simulink model "MOSSE_HDL_code_gen_final"  (Simulink 8.2)
settings: Solver=FixedStepDiscrete  SolverMode=SingleTasking  StartTime=0.0  StopTime=20*640*360  RelTol=1e-3
InitFcn:
  | %% DSPBuilder Start
  | alt_dspbuilder_update_model(bdroot)
  | %% DSPBuilder End
  | param
StopFcn:
  | % r = rcount.Data(:,:);
  | % w = wcount.Data(:,:);
  | % d = dout.Data(:,:);
  | % ir = read.Data(:,:);
  | % iw = write.Data(:,:);
  | % z = double([ir iw d r w]');
  | %logic_analyzer
values from neighbouring files (symbols this model uses):
  Gau = [4035 -3983 3832 -3589 3269 -2890 2472 -2039 1612 -1211 854 -553 ... (4096 elements, 1x4096)]    [Gauss_coeff.mat]    (also in param.m = reshape(conj(Gau'), 1, 4096))
undefined symbols (not defined in the file or in its folder): jet, psr, source_1, source_2, State_Machine, State_Transition_Table1, window_hann
libraries: allblocks_alteradspbuilder2 x182, hdldemolib x2, dspsigattribs x2, dspmtrx3 x2, visionsinks x1, visiontextngfix x1, dspvision x1
(part 3 of 3)

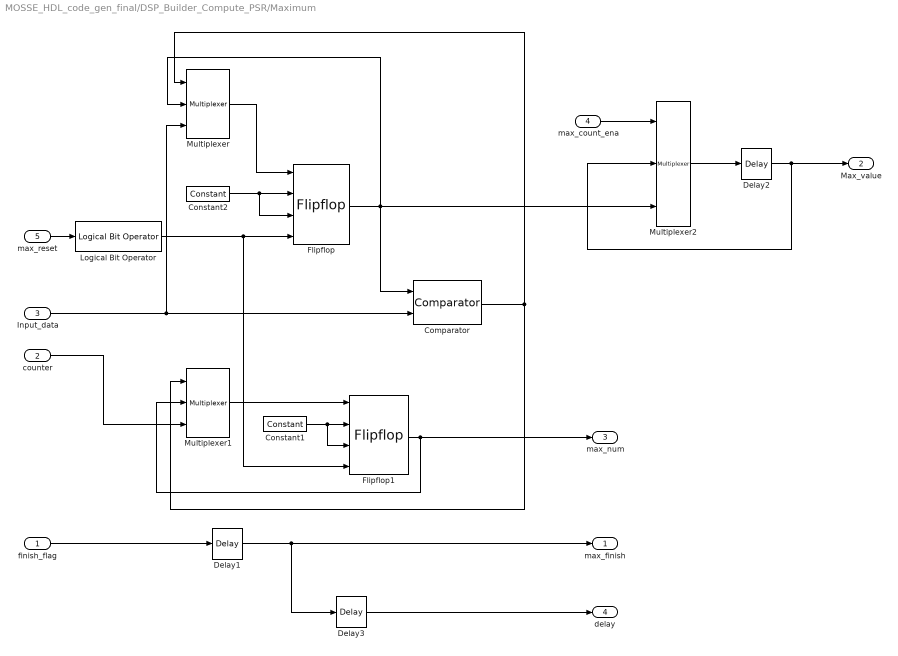
== system MOSSE_HDL_code_gen_final/DSP_Builder_Compute_PSR/Maximum ==
  finish_flag : Inport
  counter : Inport  Port=2
  Input_data : Inport  Port=3
  max_count_ena : Inport  Port=4
  max_reset : Inport  Port=5
  Comparator : allblocks_alteradspbuilder2/Comparator  direction=a < b  pipeline_display=0  allowFloatingPointOverride=on  logOutputs=off  logFile=d:\Project\AutoTracking\model\MOSSE_work\MOSSE_model\MOSSE_Final_models\tb_MOSSE_HDL_final\MOSSE%5FHDL%5Ffinal_DSP%5FBuilder%5FCompute%5FPSR_Maximum_Comparator.fixedpointlog
  Constant1 : allblocks_alteradspbuilder2/Constant  mask_cst=1  BusType=Single Bit  bwl=24  bwr=0  roundMode=Truncate  satMode=Wrap  SpecifyClock=off  allowFloatingPointOverride=on  logOutputs=off  logFile=d:\Project\AutoTracking\model\MOSSE_work\MOSSE_model\MOSSE_Final_models\tb_MOSSE_HDL_final\MOSSE%5FHDL%5Ffinal_DSP%5FBuilder%5FCompute%5FPSR_Maximum_Constant1.fixedpointlog
  Constant2 : allblocks_alteradspbuilder2/Constant  mask_cst=1  BusType=Single Bit  bwl=24  bwr=0  roundMode=Truncate  satMode=Wrap  SpecifyClock=off  allowFloatingPointOverride=on  logOutputs=off  logFile=d:\Project\AutoTracking\model\MOSSE_work\MOSSE_model\MOSSE_Final_models\tb_MOSSE_HDL_final\MOSSE%5FHDL%5Ffinal_DSP%5FBuilder%5FCompute%5FPSR_Maximum_Constant2.fixedpointlog
  Delay1 : allblocks_alteradspbuilder2/Delay  pipeline=2  pipeline_display=2  ClockPhase=1  use_ena=off  use_sclr=off  allowFloatingPointOverride=on  logOutputs=off  logFile=d:\Project\AutoTracking\model\MOSSE_work\MOSSE_model\MOSSE_Final_models\tb_MOSSE_HDL_final\MOSSE%5FHDL%5Ffinal_DSP%5FBuilder%5FCompute%5FPSR_Maximum_Delay1.fixedpointlog  use_init=off  reset_value=1
  Delay2 : allblocks_alteradspbuilder2/Delay  pipeline=1  pipeline_display=1  ClockPhase=1  use_ena=off  use_sclr=off  allowFloatingPointOverride=on  logOutputs=off  logFile=d:\Project\AutoTracking\model\MOSSE_work\MOSSE_model\MOSSE_Final_models\tb_MOSSE_HDL_final\MOSSE%5FHDL%5Ffinal_DSP%5FBuilder%5FCompute%5FPSR_Maximum_Delay2.fixedpointlog  use_init=off  reset_value=1
  Delay3 : allblocks_alteradspbuilder2/Delay  pipeline=1  pipeline_display=1  ClockPhase=1  use_ena=off  use_sclr=off  allowFloatingPointOverride=on  logOutputs=off  logFile=d:\Project\AutoTracking\model\MOSSE_work\MOSSE_model\MOSSE_Final_models\tb_MOSSE_HDL_final\MOSSE%5FHDL%5Ffinal_DSP%5FBuilder%5FCompute%5FPSR_Maximum_Delay3.fixedpointlog  use_init=off  reset_value=1
  Flipflop : allblocks_alteradspbuilder2/Flipflop  mode=DFFE  BusType=Signed Integer  bwl=16  bwr=2  pipeline_display=1
  Flipflop1 : allblocks_alteradspbuilder2/Flipflop  mode=DFFE  BusType=Signed Integer  bwl=16  bwr=2  pipeline_display=1
  Logical Bit Operator : allblocks_alteradspbuilder2/Logical Bit Operator  LogicalOperator=NOT  user_inputs=2  pipeline_display=0
  Multiplexer : allblocks_alteradspbuilder2/Multiplexer  numInputs=2  pipeline=0  oneHot=off  pipeline_display=0  use_ena=off  use_aclr=off  allowFloatingPointOverride=on  logOutputs=off  logFile=d:\Project\AutoTracking\model\MOSSE_work\MOSSE_model\MOSSE_Final_models\tb_MOSSE_HDL_final\MOSSE%5FHDL%5Ffinal_DSP%5FBuilder%5FCompute%5FPSR_Maximum_Multiplexer.fixedpointlog
  Multiplexer1 : allblocks_alteradspbuilder2/Multiplexer  numInputs=2  pipeline=0  oneHot=off  pipeline_display=0  use_ena=off  use_aclr=off  allowFloatingPointOverride=on  logOutputs=off  logFile=d:\Project\AutoTracking\model\MOSSE_work\MOSSE_model\MOSSE_Final_models\tb_MOSSE_HDL_final\MOSSE%5FHDL%5Ffinal_DSP%5FBuilder%5FCompute%5FPSR_Maximum_Multiplexer1.fixedpointlog
  Multiplexer2 : allblocks_alteradspbuilder2/Multiplexer  numInputs=2  pipeline=0  oneHot=off  pipeline_display=0  use_ena=off  use_aclr=off  allowFloatingPointOverride=on  logOutputs=off  logFile=d:\Project\AutoTracking\model\MOSSE_work\MOSSE_model\MOSSE_Final_models\tb_MOSSE_HDL_final\MOSSE%5FHDL%5Ffinal_DSP%5FBuilder%5FCompute%5FPSR_Maximum_Multiplexer2.fixedpointlog
  max_finish : Outport
  Max_value : Outport  Port=2
  max_num : Outport  Port=3
  delay : Outport  Port=4
  wires:
  Comparator/1 -> Multiplexer/1, Multiplexer1/1
  Flipflop/1 -> Comparator/1, Multiplexer2/3, Multiplexer/2
  Multiplexer/1 -> Flipflop/1
  Constant2/1 -> Flipflop/3, Flipflop/2
  Input_data/1 -> Multiplexer/3, Comparator/2
  Flipflop1/1 -> max_num/1, Multiplexer1/2
  Multiplexer1/1 -> Flipflop1/1
  Constant1/1 -> Flipflop1/3, Flipflop1/2
  counter/1 -> Multiplexer1/3
  Delay1/1 -> max_finish/1, Delay3/1
  max_count_ena/1 -> Multiplexer2/1
  Multiplexer2/1 -> Delay2/1
  Delay2/1 -> Multiplexer2/2, Max_value/1
  Delay3/1 -> delay/1
  finish_flag/1 -> Delay1/1
  Logical Bit Operator/1 -> Flipflop1/4, Flipflop/4
  max_reset/1 -> Logical Bit Operator/1

== system MOSSE_HDL_code_gen_final/DSP_Builder_Compute_PSR/Mean1 ==
  finish_flag : Inport
  Input_data : Inport  Port=2
  mean_count_ena : Inport  Port=3
  mean_reset : Inport  Port=4
  Barrel Shifter : allblocks_alteradspbuilder2/Barrel Shifter  BusType=Signed Integer  bwl=32  bwr=8  pipeline=off  infer_distance=off  distance_length=4  ShiftDirection=Shift right  use_ena=off  use_aclr=off  UseDedicatedCircuitry=off  pipeline_display=0  allowFloatingPointOverride=on  logOutputs=off  logFile=d:\Project\AutoTracking\model\MOSSE_work\MOSSE_model\MOSSE_Final_models\tb_MOSSE_HDL_final\MOSSE%5FHDL%5Ffinal_DSP%5FBuilder%5FCompute%5FPSR_Mean1_Barrel+Shifter.fixedpointlog
  Constant2 : allblocks_alteradspbuilder2/Constant  mask_cst=12  BusType=Unsigned Integer  bwl=4  bwr=0  roundMode=Truncate  satMode=Wrap  SpecifyClock=off  allowFloatingPointOverride=on  logOutputs=off  logFile=d:\Project\AutoTracking\model\MOSSE_work\MOSSE_model\MOSSE_Final_models\tb_MOSSE_HDL_final\MOSSE%5FHDL%5Ffinal_DSP%5FBuilder%5FCompute%5FPSR_Mean1_Constant2.fixedpointlog
  Delay1 : allblocks_alteradspbuilder2/Delay  pipeline=1  pipeline_display=1  ClockPhase=1  use_ena=off  use_sclr=off  allowFloatingPointOverride=on  logOutputs=off  logFile=d:\Project\AutoTracking\model\MOSSE_work\MOSSE_model\MOSSE_Final_models\tb_MOSSE_HDL_final\MOSSE%5FHDL%5Ffinal_DSP%5FBuilder%5FCompute%5FPSR_Mean1_Delay1.fixedpointlog  use_init=off  reset_value=1
  Delay2 : allblocks_alteradspbuilder2/Delay  pipeline=1  pipeline_display=1  ClockPhase=1  use_ena=off  use_sclr=off  allowFloatingPointOverride=on  logOutputs=off  logFile=d:\Project\AutoTracking\model\MOSSE_work\MOSSE_model\MOSSE_Final_models\tb_MOSSE_HDL_final\MOSSE%5FHDL%5Ffinal_DSP%5FBuilder%5FCompute%5FPSR_Mean1_Delay2.fixedpointlog  use_init=off  reset_value=1
  Multiplexer2 : allblocks_alteradspbuilder2/Multiplexer  numInputs=2  pipeline=0  oneHot=off  pipeline_display=0  use_ena=off  use_aclr=off  allowFloatingPointOverride=on  logOutputs=off  logFile=d:\Project\AutoTracking\model\MOSSE_work\MOSSE_model\MOSSE_Final_models\tb_MOSSE_HDL_final\MOSSE%5FHDL%5Ffinal_DSP%5FBuilder%5FCompute%5FPSR_Mean1_Multiplexer2.fixedpointlog
  Pipelined Adder : allblocks_alteradspbuilder2/Pipelined Adder  BusType=Signed Integer  bwl=32  bwr=0  pipeline=1  pipeline_display=1  AddSubDirection=ADD  use_cin=off  use_ovl=off  use_addsub=off  use_ena=off  use_aclr=on  or_aclr_inputs=off
  mean_finish : Outport
  mean_value : Outport  Port=2
  wires:
  Constant2/1 -> Barrel Shifter/2
  Pipelined Adder/1 -> Pipelined Adder/1, Barrel Shifter/1
  Input_data/1 -> Pipelined Adder/2
  Barrel Shifter/1 -> Multiplexer2/3
  mean_count_ena/1 -> Multiplexer2/1
  Multiplexer2/1 -> Delay2/1
  Delay2/1 -> mean_value/1, Multiplexer2/2
  finish_flag/1 -> Delay1/1
  Delay1/1 -> mean_finish/1
  mean_reset/1 -> Pipelined Adder/3

== system MOSSE_HDL_code_gen_final/DSP_Builder_Compute_PSR/Psr1 ==
  max : Inport
  mean : Inport  Port=2
  std : Inport  Port=3
  psr_count_ena : Inport  Port=4
  std_finish : Inport  Port=5
  Delay1 : allblocks_alteradspbuilder2/Delay  pipeline=1  pipeline_display=1  ClockPhase=1  use_ena=off  use_sclr=off  allowFloatingPointOverride=on  logOutputs=off  logFile=d:\Project\AutoTracking\model\MOSSE_work\MOSSE_model\MOSSE_Final_models\tb_MOSSE_HDL_final\MOSSE%5FHDL%5Ffinal_DSP%5FBuilder%5FCompute%5FPSR_Psr1_Delay1.fixedpointlog  use_init=off  reset_value=1
  Delay2 : allblocks_alteradspbuilder2/Delay  pipeline=1  pipeline_display=1  ClockPhase=1  use_ena=off  use_sclr=off  allowFloatingPointOverride=on  logOutputs=off  logFile=d:\Project\AutoTracking\model\MOSSE_work\MOSSE_model\MOSSE_Final_models\tb_MOSSE_HDL_final\MOSSE%5FHDL%5Ffinal_DSP%5FBuilder%5FCompute%5FPSR_Psr1_Delay2.fixedpointlog  use_init=off  reset_value=1
  Divider : allblocks_alteradspbuilder2/Divider  BusType=Signed Integer  bwl=32  bwr=0  pipeline=0  pipeline_display=0  use_ena=off  use_aclr=off
  Multiplexer3 : allblocks_alteradspbuilder2/Multiplexer  numInputs=2  pipeline=0  oneHot=off  pipeline_display=0  use_ena=off  use_aclr=off  allowFloatingPointOverride=on  logOutputs=off  logFile=d:\Project\AutoTracking\model\MOSSE_work\MOSSE_model\MOSSE_Final_models\tb_MOSSE_HDL_final\MOSSE%5FHDL%5Ffinal_DSP%5FBuilder%5FCompute%5FPSR_Psr1_Multiplexer3.fixedpointlog
  Pipelined Adder : allblocks_alteradspbuilder2/Pipelined Adder  BusType=Signed Integer  bwl=32  bwr=0  pipeline=0  pipeline_display=0  AddSubDirection=SUB  use_cin=off  use_ovl=off  use_addsub=off  use_ena=off  use_aclr=off  or_aclr_inputs=on
  Psr_finish : Outport
  psr : Outport  Port=2
  wires:
  Pipelined Adder/1 -> Divider/1
  Divider/1 -> Multiplexer3/3
  max/1 -> Pipelined Adder/1
  mean/1 -> Pipelined Adder/2
  std/1 -> Divider/2
  psr_count_ena/1 -> Multiplexer3/1
  Multiplexer3/1 -> Delay2/1
  Delay2/1 -> psr/1, Multiplexer3/2
  std_finish/1 -> Delay1/1
  Delay1/1 -> Psr_finish/1

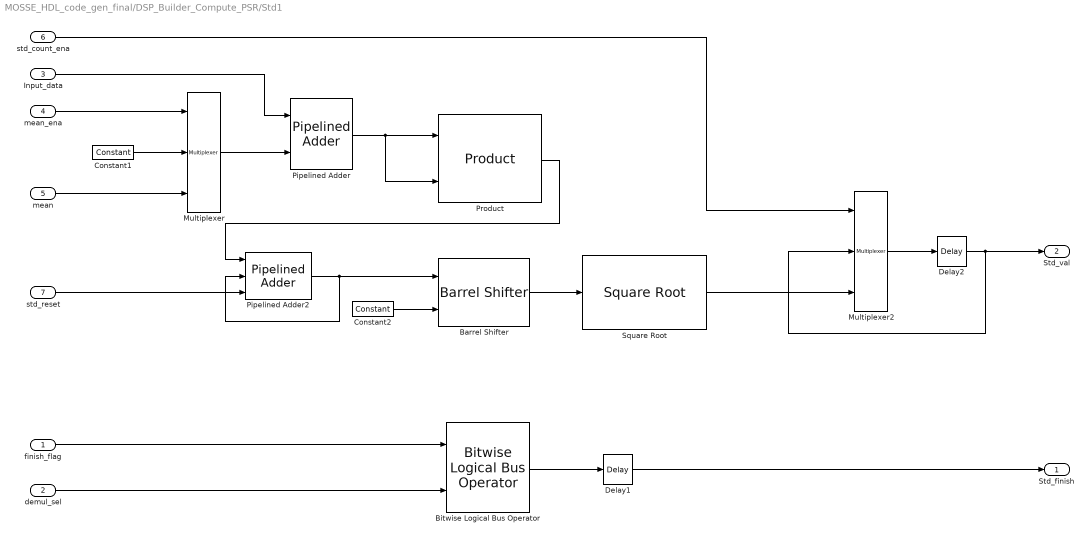
== system MOSSE_HDL_code_gen_final/DSP_Builder_Compute_PSR/Std1 ==
  finish_flag : Inport
  demul_sel : Inport  Port=2
  Input_data : Inport  Port=3
  mean_ena : Inport  Port=4
  mean : Inport  Port=5
  std_count_ena : Inport  Port=6
  std_reset : Inport  Port=7
  Barrel Shifter : allblocks_alteradspbuilder2/Barrel Shifter  BusType=Signed Integer  bwl=44  bwr=8  pipeline=off  infer_distance=off  distance_length=4  ShiftDirection=Shift right  use_ena=off  use_aclr=off  UseDedicatedCircuitry=off  pipeline_display=0  allowFloatingPointOverride=on  logOutputs=off  logFile=d:\Project\AutoTracking\model\MOSSE_work\MOSSE_model\MOSSE_Final_models\tb_MOSSE_HDL_final\MOSSE%5FHDL%5Ffinal_DSP%5FBuilder%5FCompute%5FPSR_Std1_Barrel+Shifter.fixedpointlog
  Bitwise Logical Bus Operator : allblocks_alteradspbuilder2/Bitwise Logical Bus Operator  BusType=Unsigned Integer  bwl=1  bwr=0  LogicalOperator=AND  pipeline_display=0
  Constant1 : allblocks_alteradspbuilder2/Constant  mask_cst=0  BusType=Signed Integer  bwl=32  bwr=0  roundMode=Truncate  satMode=Wrap  SpecifyClock=off  allowFloatingPointOverride=on  logOutputs=off  logFile=d:\Project\AutoTracking\model\MOSSE_work\MOSSE_model\MOSSE_Final_models\tb_MOSSE_HDL_final\MOSSE%5FHDL%5Ffinal_DSP%5FBuilder%5FCompute%5FPSR_Std1_Constant1.fixedpointlog
  Constant2 : allblocks_alteradspbuilder2/Constant  mask_cst=12  BusType=Unsigned Integer  bwl=4  bwr=0  roundMode=Truncate  satMode=Wrap  SpecifyClock=off  allowFloatingPointOverride=on  logOutputs=off  logFile=d:\Project\AutoTracking\model\MOSSE_work\MOSSE_model\MOSSE_Final_models\tb_MOSSE_HDL_final\MOSSE%5FHDL%5Ffinal_DSP%5FBuilder%5FCompute%5FPSR_Std1_Constant2.fixedpointlog
  Delay1 : allblocks_alteradspbuilder2/Delay  pipeline=1  pipeline_display=1  ClockPhase=1  use_ena=off  use_sclr=off  allowFloatingPointOverride=on  logOutputs=off  logFile=d:\Project\AutoTracking\model\MOSSE_work\MOSSE_model\MOSSE_Final_models\tb_MOSSE_HDL_final\MOSSE%5FHDL%5Ffinal_DSP%5FBuilder%5FCompute%5FPSR_Std1_Delay1.fixedpointlog  use_init=off  reset_value=1
  Delay2 : allblocks_alteradspbuilder2/Delay  pipeline=1  pipeline_display=1  ClockPhase=1  use_ena=off  use_sclr=off  allowFloatingPointOverride=on  logOutputs=off  logFile=d:\Project\AutoTracking\model\MOSSE_work\MOSSE_model\MOSSE_Final_models\tb_MOSSE_HDL_final\MOSSE%5FHDL%5Ffinal_DSP%5FBuilder%5FCompute%5FPSR_Std1_Delay2.fixedpointlog  use_init=off  reset_value=1
  Multiplexer : allblocks_alteradspbuilder2/Multiplexer  numInputs=2  pipeline=0  oneHot=off  pipeline_display=0  use_ena=off  use_aclr=off  allowFloatingPointOverride=on  logOutputs=off  logFile=d:\Project\AutoTracking\model\MOSSE_work\MOSSE_model\MOSSE_Final_models\tb_MOSSE_HDL_final\MOSSE%5FHDL%5Ffinal_DSP%5FBuilder%5FCompute%5FPSR_Std1_Multiplexer.fixedpointlog
  Multiplexer2 : allblocks_alteradspbuilder2/Multiplexer  numInputs=2  pipeline=0  oneHot=off  pipeline_display=0  use_ena=off  use_aclr=off  allowFloatingPointOverride=on  logOutputs=off  logFile=d:\Project\AutoTracking\model\MOSSE_work\MOSSE_model\MOSSE_Final_models\tb_MOSSE_HDL_final\MOSSE%5FHDL%5Ffinal_DSP%5FBuilder%5FCompute%5FPSR_Std1_Multiplexer2.fixedpointlog
  Pipelined Adder : allblocks_alteradspbuilder2/Pipelined Adder  BusType=Signed Integer  bwl=32  bwr=0  pipeline=0  pipeline_display=0  AddSubDirection=SUB  use_cin=off  use_ovl=off  use_addsub=off  use_ena=off  use_aclr=off  or_aclr_inputs=on
  Pipelined Adder2 : allblocks_alteradspbuilder2/Pipelined Adder  BusType=Signed Integer  bwl=44  bwr=0  pipeline=1  pipeline_display=1  AddSubDirection=ADD  use_cin=off  use_ovl=off  use_addsub=off  use_ena=off  use_aclr=on  or_aclr_inputs=off
  Product : allblocks_alteradspbuilder2/Product  BusType=Signed Integer  bwl=32  bwr=0  pipeline=0  pipeline_display=0  phase_selection=1  use_ena=off  use_aclr=off  UseLPM=off  UseDedicatedCircuitry=on  allowFloatingPointOverride=on  logOutputs=off  logFile=d:\Project\AutoTracking\model\MOSSE_work\MOSSE_model\MOSSE_Final_models\tb_MOSSE_HDL_final\MOSSE%5FHDL%5Ffinal_DSP%5FBuilder%5FCompute%5FPSR_Std1_Product.fixedpointlog
  Square Root : allblocks_alteradspbuilder2/Square Root  BusType=Unsigned Integer  bwl=44  bwr=0  pipeline=0  pipeline_display=0  use_remain=off  use_ena=off  use_aclr=off
  Std_finish : Outport
  Std_val : Outport  Port=2
  wires:
  Pipelined Adder/1 -> Product/2, Product/1
  Product/1 -> Pipelined Adder2/1
  Constant2/1 -> Barrel Shifter/2
  Pipelined Adder2/1 -> Pipelined Adder2/2, Barrel Shifter/1
  Barrel Shifter/1 -> Square Root/1
  Square Root/1 -> Multiplexer2/3
  Input_data/1 -> Pipelined Adder/1
  demul_sel/1 -> Bitwise Logical Bus Operator/2
  finish_flag/1 -> Bitwise Logical Bus Operator/1
  Delay1/1 -> Std_finish/1
  Constant1/1 -> Multiplexer/2
  mean_ena/1 -> Multiplexer/1
  mean/1 -> Multiplexer/3
  Multiplexer/1 -> Pipelined Adder/2
  std_count_ena/1 -> Multiplexer2/1
  Multiplexer2/1 -> Delay2/1
  Delay2/1 -> Std_val/1, Multiplexer2/2
  Bitwise Logical Bus Operator/1 -> Delay1/1
  std_reset/1 -> Pipelined Adder2/3

== system MOSSE_HDL_code_gen_final/DSP_Builder_Compute_PSR/Vals_gen ==
  count_ena : Inport
  counter : Inport  Port=2
  demul_sel : Inport  Port=3
  Constant2 : allblocks_alteradspbuilder2/Constant  mask_cst=0  BusType=Single Bit  bwl=16  bwr=0  roundMode=Truncate  satMode=Wrap  SpecifyClock=off  allowFloatingPointOverride=on  logOutputs=off  logFile=d:\Project\AutoTracking\model\MOSSE_work\MOSSE_model\MOSSE_Final_models\tb_MOSSE_HDL_final\MOSSE%5FHDL%5Ffinal_DSP%5FBuilder%5FCompute%5FPSR_Vals%5Fgen_Constant2.fixedpointlog
  Demultiplexer : allblocks_alteradspbuilder2/Demultiplexer  numOutputs=2  pipeline_display=1  use_ena=off  use_sclr=off  allowFloatingPointOverride=on  logOutputs=off  logFile=d:\Project\AutoTracking\model\MOSSE_work\MOSSE_model\MOSSE_Final_models\tb_MOSSE_HDL_final\MOSSE%5FHDL%5Ffinal_DSP%5FBuilder%5FCompute%5FPSR_Vals%5Fgen_Demultiplexer%3A%3Aq.fixedpointlog,d:\Project\AutoTracking\model\MOSSE_work\MOSSE_model\MOSSE_Final_models\tb_MOSSE_HDL_final\MOSSE%5FHDL%5Ffinal_DSP%5FBuilder%5FCompute%5FPSR_Vals%5Fgen_Demultiplexer%3A%3Aq.fixedpointlog,
  Multiplexer : allblocks_alteradspbuilder2/Multiplexer  numInputs=2  pipeline=0  oneHot=off  pipeline_display=0  use_ena=off  use_aclr=off  allowFloatingPointOverride=on  logOutputs=off  logFile=d:\Project\AutoTracking\model\MOSSE_work\MOSSE_model\MOSSE_Final_models\tb_MOSSE_HDL_final\MOSSE%5FHDL%5Ffinal_DSP%5FBuilder%5FCompute%5FPSR_Vals%5Fgen_Multiplexer.fixedpointlog
  1_channel : Outport
  2_channel : Outport  Port=2
  wires:
  Multiplexer/1 -> Demultiplexer/1
  Demultiplexer/1 -> 1_channel/1
  Demultiplexer/2 -> 2_channel/1
  demul_sel/1 -> Demultiplexer/2
  Constant2/1 -> Multiplexer/2
  counter/1 -> Multiplexer/3
  count_ena/1 -> Multiplexer/1

== system MOSSE_HDL_code_gen_final/DSP_Builder_Mult_complex/Gauss_table ==
  rst : Inport
  enb : Inport  Port=2
  Counter : allblocks_alteradspbuilder2/Counter  BusType=Unsigned Integer  bwl=12  bwr=0  use_modulo=off  modulo=255  SpecifyClock=off  direction=Increment  use_sload=off  use_sset=off  svalue=1  use_clk_ena=off  use_ena=on  use_sclr=on  pipeline_display=1
  ROM : allblocks_alteradspbuilder2/ROM  numwords=4096  BusType=Signed Integer  bwl=16  bwr=0  memory_type=AUTO  ram_type=ROM  initialization=From MATLAB array  init_file=input.hex  init_array=imag(Gau)  register_outputs=off  use_ena=off  ClockPhase=1  pipeline_display=1  allowFloatingPointOverride=on  logOutputs=off  logFile=E:\Project\AutoTracking\AutoTrack\Model\MOSSE_algorithm\MOSSE_simulink\tb_MOSSE_HDL_code_gen_final\MOSSE%5FHDL%5Fcode%5Fgen%5Ffinal_DSP%5FBuilder%5FMult%5Fcomplex_Gauss%5Ftable_ROM.fixedpointlog  enable_runtime_mod=off  instance_name=AAAA
  ROM1 : allblocks_alteradspbuilder2/ROM  numwords=4096  BusType=Signed Integer  bwl=16  bwr=0  memory_type=AUTO  ram_type=ROM  initialization=From MATLAB array  init_file=input.hex  init_array=real(Gau)  register_outputs=off  use_ena=off  ClockPhase=1  pipeline_display=1  allowFloatingPointOverride=on  logOutputs=off  logFile=E:\Project\AutoTracking\AutoTrack\Model\MOSSE_algorithm\MOSSE_simulink\tb_MOSSE_HDL_code_gen_final\MOSSE%5FHDL%5Fcode%5Fgen%5Ffinal_DSP%5FBuilder%5FMult%5Fcomplex_Gauss%5Ftable_ROM1.fixedpointlog  enable_runtime_mod=off  instance_name=AAAA
  Coeff_real : Outport
  Coeff_imag : Outport  Port=2
  wires:
  Counter/1 -> ROM/1, ROM1/1
  ROM1/1 -> Coeff_real/1
  ROM/1 -> Coeff_imag/1
  rst/1 -> Counter/2
  enb/1 -> Counter/1

== system MOSSE_HDL_code_gen_final/Source/source_1 ==
  In1 : Inport
  Enable : EnablePort
  source_1 : LookupNDDirect  NumberOfTableDimensions=1  Table=source_1  TableDataTypeStr=int16
  Out1 : Outport
  wires:
  source_1/1 -> Out1/1
  In1/1 -> source_1/1

== system MOSSE_HDL_code_gen_final/Source/source_2 ==
  In1 : Inport
  Enable : EnablePort
  source_2 : LookupNDDirect  NumberOfTableDimensions=1  Table=source_2  TableDataTypeStr=int16
  Out1 : Outport
  wires:
  source_2/1 -> Out1/1
  In1/1 -> source_2/1

== system MOSSE_HDL_code_gen_final/Video_TestBench1/Write_control_subsys ==
  addr_x : Inport
  addr_y : Inport  Port=2
  dx : Inport  Port=3
  dy : Inport  Port=4
  x_init : Inport  Port=5
  y_init : Inport  Port=6
  comp_shift_finish : Inport  Port=7
  Write_control_STM : State Transition Table  TreatAsAtomicUnit=on
  x_coord : Outport
  y_coord : Outport  Port=2
  enable_write : Outport  Port=3
  wires:
  x_init/1 -> Write_control_STM/6(x_init)
  y_init/1 -> Write_control_STM/7(y_init)
  dx/1 -> Write_control_STM/3(dx)
  dy/1 -> Write_control_STM/4(dy)
  Write_control_STM/1(x_coord) -> x_coord/1
  Write_control_STM/3(enable_write) -> enable_write/1
  Write_control_STM/2(y_coord) -> y_coord/1
  comp_shift_finish/1 -> Write_control_STM/5(comp_shift_finish)
  addr_x/1 -> Write_control_STM/1(addr_x)
  addr_y/1 -> Write_control_STM/2(addr_y)

== system MOSSE_HDL_code_gen_final/Video_TestBench1/deserialize1 ==
  serialin : Inport
  Buffer : Buffer  N=640*360  TreatMby1Signals=One channel
  Convert 1-D to 2-D : dspsigattribs/Convert 1-D to 2-D  M=640  N=360  frameBasedOut=off
  Frame Conversion : FrameConversion  OutFrame=Sample-based
  Transpose : dspmtrx3/Transpose  Hermitian=off  overflowFlag=on
  imgout : Outport
  wires:
  Buffer/1 -> Frame Conversion/1
  serialin/1 -> Buffer/1
  Convert 1-D to 2-D/1 -> Transpose/1
  Frame Conversion/1 -> Convert 1-D to 2-D/1
  Transpose/1 -> imgout/1

== system MOSSE_HDL_code_gen_final/Video_TestBench1/serialize ==
  img : Inport
  Convert 2-D to 1-D : dspsigattribs/Convert 2-D to 1-D
  Frame Conversion : FrameConversion
  Transpose : dspmtrx3/Transpose  Hermitian=off  overflowFlag=on
  Unbuffer : Unbuffer  SampleBasedProcessing=Same as frame based
  serial : Outport  SampleTime=1
  wires:
  Convert 2-D to 1-D/1 -> Frame Conversion/1
  img/1 -> Transpose/1
  Transpose/1 -> Convert 2-D to 1-D/1
  Frame Conversion/1 -> Unbuffer/1
  Unbuffer/1 -> serial/1

== stateflow chart Source/State Transition Table ==
  state state2
    entry:
    enable_write = false;
  state state1
    entry:
    enable_write = false;
  state state3
    entry:
    enable_write = true;
  state state4
    entry:
    enable_write = false;
  state1 -> (junction 27) [order 2]
  (default) -> state1
  (junction 27) -> state1
  state1 -> state2 [order 1] : {temp = 0;
      | count = 0;}
  state2 -> (junction 28) [order 2]
  (junction 28) -> state2
  (junction 29) -> state2
  (junction 32) -> (junction 29)
  state2 -> state3 [order 1] : [address == 99541 + temp*640]
  state3 -> (junction 30) [order 1] : [count ~= 127]
      | {count = count + 1;}
  (junction 30) -> state3
  state3 -> state4 [order 2] : {temp = temp + 1;
      |  count = 0;}
  state4 -> (junction 31) [order 2] : {temp = 0;}
  (junction 31) -> state4
  state4 -> (junction 32) [order 1] : [temp ~= 128]
  data: enable_write output boolean; address input uint32; temp local double; count local double

== stateflow chart Video_TestBench1/Write_control_subsys/Write_control_STM ==
  settings: executeAtInitialization=1
  state state2
    % Автомат управления сигналом записи кадра в память
    entry:
    x_coord = x;
    y_coord = y;
    enable_write = false;
  state state1
    % Условия по-умолчанию
    entry:
    enable_write = false;
    x_coord = fi(0,0,10,0);
    y_coord = fi(0,0,9,0);
  state state3
    entry:
    enable_write = true;
  state state4
    entry:
    enable_write = false;
  state state5
    % Кадр записан
    % Обновление значений смещения
    entry:
    enable_write = false;
  state state6
    % Обновление значений координат
    entry:
    enable_write = false;
  state1 -> (junction 102) [order 2]
  (default) -> state1
  (junction 102) -> state1
  state1 -> state2 [order 1] : {count = fi(0,0,8,0);
      | x = fi(x_init,0,10,0);
      | y = fi(y_init,0,9,0);
      | temp_x = fi(x + 128,0,10,0);
      | temp_y = fi(y + count,0,9,0);
      | Dx = int8(0);
      | Dy = int8(0);}
  state2 -> (junction 103) [order 3]
  (junction 103) -> state2
  (junction 104) -> state2
  state2 -> (junction 105) [order 2] : [comp_shift_finish == true && count == 0]
  (junction 107) -> (junction 104)
  (junction 105) -> (junction 109)
  state2 -> state3 [order 1] : [addr_x == x && addr_y == temp_y && comp_shift_finish == false]
  state3 -> (junction 106) [order 1] : [addr_x ~= temp_x]
  (junction 106) -> state3
  state3 -> state4 [order 2] : {count = fi(count + 1,0,8,0);
      | temp_y = fi(y + count,0,9,0);}
  state4 -> (junction 107) [order 1] : [count ~= 128]
  (junction 111) -> (junction 107)
  state4 -> state5 [order 2] : {count = fi(0,0,8,0);}
  state5 -> (junction 108) [order 2]
  (junction 108) -> state5
  (junction 109) -> state5
  state5 -> state6 [order 1] : {Dx = dx;
      | Dy = dy;}
  state6 -> (junction 110) [order 2]
  (junction 110) -> state6
  state6 -> (junction 111) [order 1] : {x = fi(x + Dx,0,10,0);
      | y = fi(y + Dy,0,9,0);
      | temp_x = fi(x + 128,0,10,0);
      | temp_y = fi(y + count,0,9,0);}
  (junction 112) -> state6
  data: x_coord output fixdt(0,10,0); y_coord output fixdt(0,9,0); addr_x input fixdt(0,10,0); count local fixdt(0,8,0); x local fixdt(0,10,0); addr_y input fixdt(0,9,0); y local fixdt(0,9,0); dx input int8; dy input int8; Dx local int8; Dy local int8; temp_x local fixdt(0,10,0); temp_y local fixdt(0,9,0); enable_write output boolean; comp_shift_finish input boolean; x_init input uint16; y_init input uint16

== matlab function Video_TestBench1/Transpone Counter ==
  data: X output fixdt(0,10,0); clear input boolean; en input boolean; Y output fixdt(0,9,0)
function [X, Y]  = count(clear, en)

%result_nt = numerictype(0,12,0);
col_nt = numerictype(0,10,0);
row_nt = numerictype(0,9,0);

result_fm = fimath('OverflowMode', 'saturate', 'RoundMode', 'floor');
m = fi(640, 0,10,0, result_fm);
n = fi(360, 0,9,0, result_fm);
% persistent count_reg 
persistent column row

% if isempty(count_reg)
%     count_reg = fi(0, result_nt, result_fm);
% end

if isempty(column)
    column = fi(0, col_nt, result_fm);
end

if isempty(row)
    row = fi(0, row_nt, result_fm);
end

if clear
    row = fi(0, row_nt, result_fm);
    column = fi(0, col_nt, result_fm);
    % count_reg = fi(0, result_nt, result_fm);
elseif en
     
     if (column == (m-1))
         if(row ~= (n-1))
             inc_r = row + fi(1, row_nt, result_fm);
             row = fi(inc_r, row_nt, result_fm);
         else row = fi(0, row_nt, result_fm);
             
         end
         column = fi(0, col_nt, result_fm);
     else
         inc_c = column + fi(1, col_nt, result_fm);
         column = fi(inc_c, col_nt, result_fm);
     end
     %count_reg = fi(column*n + row, result_nt, result_fm);
end

X = column;
Y = row;
% count = count_reg;

end
